simulink model "AFEC_model"  (R2024a)
settings: Solver=FixedStepAuto  StartTime=0.0  StopTime=7  FixedStep=1e-5  RelTol=1e-3
values from neighbouring files (symbols this model uses):
  C1 = 750e-6    (= 0.00075)    [scriptafec11.m]
  ka = Vdcref/2    (= 378.5)    [scriptafec11.m]
  kii_1 = 2*pi*fbi*r/ka    (= 0.014940202844)    [scriptafec11.m]
  kiw_1 = kpw_1 / (a_l^2 * tau_1l)    [scriptafec11.m]
  kpi_1 = 2*pi*fbi*l/ka    (= 0.015936216367)    [scriptafec11.m]
  kpw_1 = C1 / kl / a_l / tau_1l    [scriptafec11.m]
  l = 4.8e-3    (= 0.0048)    [scriptafec11.m]
  r = 0.0045    [scriptafec11.m]
  t_c = 1.5    [scriptafec11.m]
  t_pll = 1.3    [scriptafec11.m]
  t_precharge = 1    [scriptafec11.m]
  t_v = 1.75    [scriptafec11.m]
  tau_fl = 1 / 200    (= 0.005)    [scriptafec11.m]
  Vdcref = 757    [scriptafec11.m]
libraries: spsVoltageMeasurementLib x8, spsCurrentMeasurementLib x7, spsIGBTDiodeLib x6, spsSeriesRLCBranchLib x3, spsFirstOrderFilterLib x3, spsThreePhaseSeriesRLCBranchLib x2, spsControlledVoltageSourceLib x1, spsTriangleGeneratorLib x1, spsThreePhaseBreakerLib x1, spsThreePhaseSourceLib x1, sps_lib x1
settings Model: Creator=SSP Family  LastModifiedBy=khush
settings SolverCC: ZeroCrossAlgorithm=Adaptive
settings DebuggingCC: MaskedZcDiagnostic=none  IgnoredZcDiagnostic=none

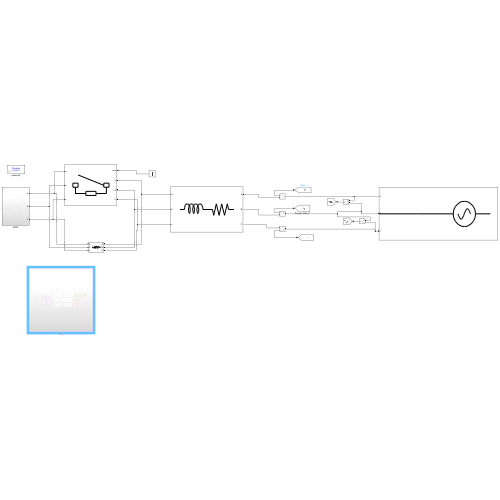
[thumbnail: Simulink's stored preview of the top-level diagram]
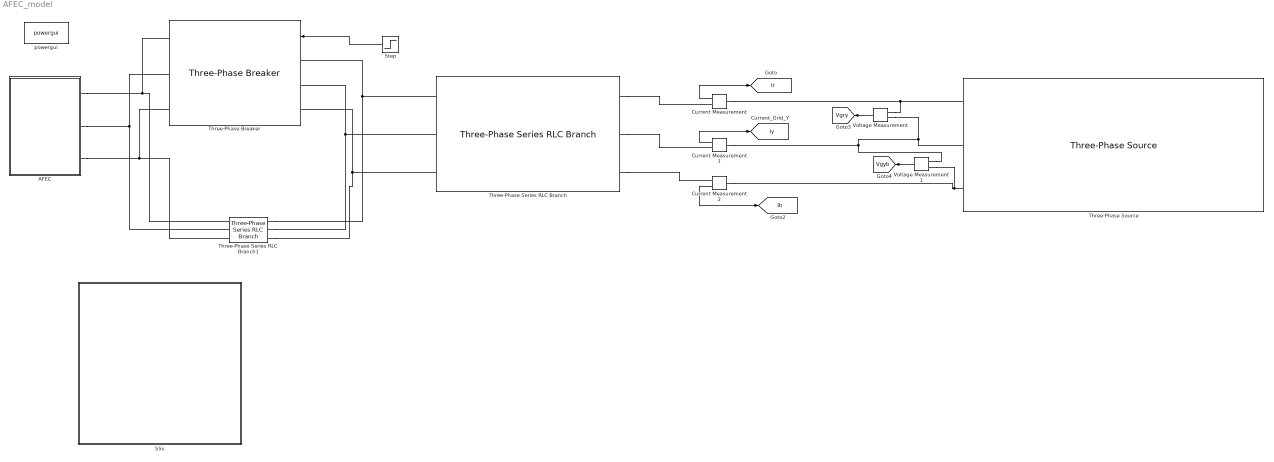
== system AFEC_model ==
  AFEC : Subsystem
  Current Measurement : spsCurrentMeasurementLib/Current Measurement  PhasorSimulation=off  OutputType=Complex  PSBequivalent=0
  Current Measurement1 : spsCurrentMeasurementLib/Current Measurement  PhasorSimulation=off  OutputType=Complex  PSBequivalent=0
  Current Measurement2 : spsCurrentMeasurementLib/Current Measurement  PhasorSimulation=off  OutputType=Complex  PSBequivalent=0
  SSs : Subsystem
  Step : Step  Time=t_precharge  SampleTime=0
  Three-Phase Series RLC Branch : spsThreePhaseSeriesRLCBranchLib/Three-Phase Series RLC Branch  LConnTagsString=A|B|C  RConnTagsString=A|B|C  BranchType=RL  Resistance=r  Inductance=l  Capacitance=1e-6  Measurements=None
  Three-Phase Series RLC Branch1 : spsThreePhaseSeriesRLCBranchLib/Three-Phase Series RLC Branch  LConnTagsString=A|B|C  RConnTagsString=A|B|C  BranchType=R  Resistance=2e3  Inductance=1e-3  Capacitance=1e-6  Measurements=None
  Three-Phase Breaker : spsThreePhaseBreakerLib/Three-Phase Breaker  InitialState=open  SwitchA=on  SwitchB=on  SwitchC=on  SwitchTimes="[1/60  5/60]"  External=on  BreakerResistance=0.01  SnubberResistance=1e6  SnubberCapacitance=inf  Measurements=None
  Three-Phase Source : spsThreePhaseSourceLib/Three-Phase Source  InternalConnection=Y  VoltagePhases=off  Voltage=400/sqrt(3)  PhaseAngle=0  Voltage_phases=[25e3 25e3 25e3]/sqrt(3)  PhaseAngles_phases=[0 -120 +120]  Frequency=50  NonIdealSource=off  SpecifyImpedance=off  Resistance=0  Inductance=0  ShortCircuitLevel=100e6  BaseVoltage=25e3  XRratio=7  BusType=swing  Pref=10e3  Qref=0  Prefabc=[10e3, 10e3, 10e3]  Qrefabc=[0, 0, 0]  Qmin=-inf  Qmax=inf
  Voltage Measurement : spsVoltageMeasurementLib/Voltage Measurement  PhasorSimulation=off  OutputType=Complex  PSBequivalent=0
  Voltage Measurement1 : spsVoltageMeasurementLib/Voltage Measurement  PhasorSimulation=off  OutputType=Complex  PSBequivalent=0
  powergui : sps_lib/powergui  Priority=1  SimulationMode=Discrete  SampleTime=1e-5  frequency=60  Iterations=50  frequencyindice=0  Pbase=100e6  ErrMax=1e-4  UnitsV=kV  UnitsW=MW  buscounter=0  FunctionMessages=off  echomessages=off  EnableUseOfTLC=off  CurrentSourceSwitches=off  DisableSnubberDevices=off  DisableRonSwitches=off  DisableVfSwitches=off  DisplayEquations=off  AutomaticDiscreteSolvers=off  SolverType=Tustin/Backward Euler (TBE)  Interpol=off  ExternalGateDelay=off  methode=off  Ts=100  x0status=blocks  SPID=on  SwTol=0  HookPort=off  NonlinearTolerance=1e-4  nMaxIteration=100  ContinueOnMaxIteration=off  RestoreLinks=warning  ResistiveCurrentMeasurement=off  Frange=[0:2:500]  Ylog=off  Xlog=on  ShowGrid=off  save=off  variable=ZData  structure=0  ZoomFFT=off  StartTime=0.0  cycles=1  DisplayStyle=1  fundamental=60  FreqAxis=off  MaxFrequency=1000  frequencyindicesteady=1  RmsSteady=1  display=off
  tag scope: Ib=global, Ir=global, Iy=global, Vgry=global, Vgyb=global
  wires:
  Current Measurement2/1 -> [Ib]
  Voltage Measurement/1 -> [Vgry]
  Voltage Measurement1/1 -> [Vgyb]
  Step/1 -> Three-Phase Breaker/1
  Current Measurement/1 -> [Ir]
  Current Measurement1/1 -> [Iy]
  connections:
  Current Measurement/LConn1 -- Three-Phase Source/RConn1 -- Voltage Measurement/LConn1
  Voltage Measurement1/LConn1 -- Voltage Measurement/LConn2 -- Three-Phase Source/RConn2 -- Current Measurement1/LConn1
  Voltage Measurement1/LConn2 -- Current Measurement2/LConn1 -- Three-Phase Source/RConn3
  Three-Phase Series RLC Branch1/LConn2 -- Three-Phase Series RLC Branch/RConn2 -- Three-Phase Breaker/LConn2
  Three-Phase Series RLC Branch1/LConn1 -- Three-Phase Series RLC Branch/RConn1 -- Three-Phase Breaker/LConn1
  Three-Phase Breaker/RConn1 -- Three-Phase Series RLC Branch1/RConn1 -- AFEC/LConn1
  Three-Phase Series RLC Branch1/LConn3 -- Three-Phase Series RLC Branch/RConn3 -- Three-Phase Breaker/LConn3
  Three-Phase Breaker/RConn3 -- Three-Phase Series RLC Branch1/RConn3 -- AFEC/LConn3
  Three-Phase Series RLC Branch1/RConn2 -- AFEC/LConn2 -- Three-Phase Breaker/RConn2
  Three-Phase Series RLC Branch/LConn1 -- Current Measurement/RConn1
  Three-Phase Series RLC Branch/LConn2 -- Current Measurement1/RConn1
  Three-Phase Series RLC Branch/LConn3 -- Current Measurement2/RConn1

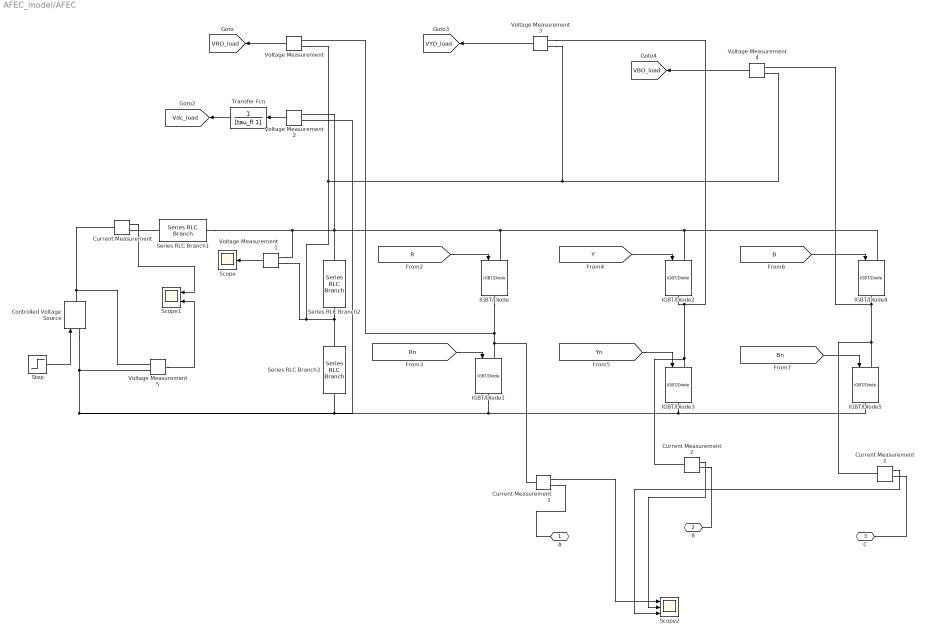
== system AFEC_model/AFEC ==
  Controlled Voltage Source : spsControlledVoltageSourceLib/Controlled Voltage Source  Initialize=on  Source_Type=DC  Amplitude=800  Phase=0  Frequency=0  Measurements=None
  Current Measurement{,1..3} (4 alike) : spsCurrentMeasurementLib/Current Measurement  PhasorSimulation=off  OutputType=Complex  PSBequivalent=0
  IGBT/Diode{,1..5} (6 alike) : spsIGBTDiodeLib/IGBT//Diode  Ron=1e-3  Rs=1e5  Cs=inf  Measurements=off
  Scope : Scope
  Scope1 : Scope  NumInputPorts=2
  Scope2 : Scope  NumInputPorts=3
  Series RLC Branch1 : spsSeriesRLCBranchLib/Series RLC Branch  LConnTagsString=__new0  RConnTagsString=__new0  BranchType=R  Resistance=10  Inductance=1e-3  SetiL0=off  InitialCurrent=0  Capacitance=1e-6  Setx0=off  InitialVoltage=0  Measurements=None
  Series RLC Branch2 : spsSeriesRLCBranchLib/Series RLC Branch  LConnTagsString=__new0  RConnTagsString=__new0  BranchType=C  Resistance=1  Inductance=1e-3  SetiL0=off  InitialCurrent=0  Capacitance=C1  Setx0=off  InitialVoltage=0  Measurements=None
  Series RLC Branch3 : spsSeriesRLCBranchLib/Series RLC Branch  LConnTagsString=__new0  RConnTagsString=__new0  BranchType=C  Resistance=1  Inductance=1e-3  SetiL0=off  InitialCurrent=0  Capacitance=C1  Setx0=off  InitialVoltage=0  Measurements=None
  Step : Step  After=800  SampleTime=0
  Transfer Fcn : TransferFcn  Denominator=[tau_fl 1]
  Voltage Measurement{,1..5} (6 alike) : spsVoltageMeasurementLib/Voltage Measurement  PhasorSimulation=off  OutputType=Complex  PSBequivalent=0
  A : PMIOPort  Side=Left
  B : PMIOPort  Port=2  Side=Left
  C : PMIOPort  Port=3  Side=Left
  tag scope: VBO_load=global, VRO_load=global, VYO_load=global, Vdc_load=global
  wires:
  Voltage Measurement4/1 -> [VBO_load]
  [Bn] -> IGBT/Diode5/1
  Voltage Measurement3/1 -> [VYO_load]
  Transfer Fcn/1 -> [Vdc_load]
  [B] -> IGBT/Diode4/1
  Voltage Measurement/1 -> [VRO_load]
  [Y] -> IGBT/Diode2/1
  Voltage Measurement2/1 -> Transfer Fcn/1
  [Rn] -> IGBT/Diode1/1
  [Yn] -> IGBT/Diode3/1
  [R] -> IGBT/Diode/1
  Step/1 -> Controlled Voltage Source/1
  Voltage Measurement1/1 -> Scope/1
  Voltage Measurement5/1 -> Scope1/2
  Current Measurement/1 -> Scope1/1
  Current Measurement1/1 -> Scope2/1
  Current Measurement2/1 -> Scope2/2
  Current Measurement3/1 -> Scope2/3
  connections:
  IGBT/Diode2/LConn1 -- Voltage Measurement1/LConn1 -- Series RLC Branch1/RConn1 -- Series RLC Branch2/LConn1 -- Voltage Measurement2/LConn1 -- IGBT/Diode/LConn1 -- IGBT/Diode4/LConn1
  IGBT/Diode/RConn1 -- Current Measurement1/LConn1 -- IGBT/Diode1/LConn1 -- Voltage Measurement/LConn1
  IGBT/Diode3/RConn1 -- IGBT/Diode5/RConn1 -- IGBT/Diode1/RConn1 -- Series RLC Branch3/RConn1 -- Controlled Voltage Source/LConn1 -- Voltage Measurement5/LConn2 -- Voltage Measurement2/LConn2
  IGBT/Diode2/RConn1 -- Voltage Measurement3/LConn1 -- Current Measurement2/LConn1 -- IGBT/Diode3/LConn1
  Voltage Measurement/LConn2 -- Voltage Measurement4/LConn2 -- Voltage Measurement3/LConn2 -- Voltage Measurement1/LConn2 -- Series RLC Branch2/RConn1 -- Series RLC Branch3/LConn1
  Controlled Voltage Source/RConn1 -- Current Measurement/LConn1 -- Voltage Measurement5/LConn1
  Current Measurement/RConn1 -- Series RLC Branch1/LConn1
  Voltage Measurement4/LConn1 -- Current Measurement3/LConn1 -- IGBT/Diode5/LConn1 -- IGBT/Diode4/RConn1
  Current Measurement1/RConn1 -- A/RConn1
  Current Measurement2/RConn1 -- B/RConn1
  Current Measurement3/RConn1 -- C/RConn1

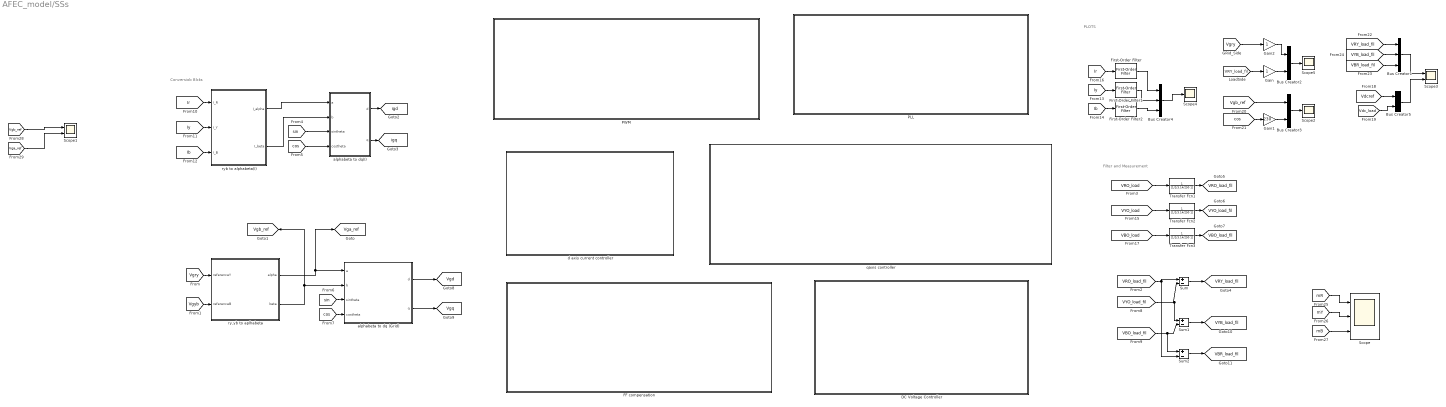
== system AFEC_model/SSs ==
  note: Conversiob Blcks
  note: PLOTS
  note: Filter and Measurement
  Bus Creator1 : BusCreator  Inputs=3
  Bus Creator2 : BusCreator  Inputs=2
  Bus Creator3 : BusCreator  Inputs=2
  Bus Creator4 : BusCreator  Inputs=3
  Bus Creator5 : BusCreator  Inputs=2
  DC Voltage Controller : Subsystem
  FF compensation : Subsystem
  First-Order Filter : spsFirstOrderFilterLib/First-Order Filter  FilterType=Lowpass  Tc=1e-3  Ts=0  Initialize=off  Vac_Init=[0, 0, 60]  Vdc_Init=0  PlotResponse=off  FreqRange="[0,  200,  1]"
  First-Order Filter1 : spsFirstOrderFilterLib/First-Order Filter  FilterType=Lowpass  Tc=10e-3  Ts=0  Initialize=off  Vac_Init=[0, 0, 60]  Vdc_Init=0  PlotResponse=off  FreqRange="[0,  200,  1]"
  First-Order Filter2 : spsFirstOrderFilterLib/First-Order Filter  FilterType=Lowpass  Tc=10e-3  Ts=0  Initialize=off  Vac_Init=[0, 0, 60]  Vdc_Init=0  PlotResponse=off  FreqRange="[0,  200,  1]"
  Gain : Gain
  Gain1 : Gain  Gain=230
  Gain2 : Gain
  PLL : Subsystem
  PWM : Subsystem
  Scope : Scope  NumInputPorts=3
  Scope1 : Scope  NumInputPorts=2
  Scope2 : Scope
  Scope3 : Scope  NumInputPorts=2
  Scope4 : Scope
  Scope5 : Scope
  Sum : Sum  Inputs=+-
  Sum1 : Sum  Inputs=+-
  Sum2 : Sum  Inputs=+-
  Transfer Fcn1 : TransferFcn  Denominator=[1/2/3.14/250 1]
  Transfer Fcn2 : TransferFcn  Denominator=[1/2/3.14/250 1]
  Transfer Fcn3 : TransferFcn  Denominator=[1/2/3.14/250 1]
  alphabeta to dq (Grid) : MATLAB Function  TreatAsAtomicUnit=on
  alphabeta to dq(I) : MATLAB Function  TreatAsAtomicUnit=on
  d axis current controller : Subsystem
  qaxis controller : Subsystem
  ry,yb to aplhabeta : MATLAB Function  TreatAsAtomicUnit=on
  ryb to alphabeta(I) : MATLAB Function  TreatAsAtomicUnit=on
  tag scope: VBO_load_fil=global, VBR_load_fil=global, VRO_load_fil=global, VRY_load_fil=global, VYB_load_fil=global, VYO_load_fil=global, Vga_ref=global, Vgb_ref=global, Vgd=global, Vgq=global, igd=global, igq=global
  wires:
  ry,yb to aplhabeta/2(beta) -> [Vgb_ref], alphabeta to dq (Grid)/2(b)
  [Ib] -> ryb to alphabeta(I)/3(I_B)
  ry,yb to aplhabeta/1(alpha) -> [Vga_ref], alphabeta to dq (Grid)/1(a)
  ryb to alphabeta(I)/1(I_alpha) -> alphabeta to dq(I)/1(a)
  [cos] -> alphabeta to dq (Grid)/4(costheta)
  [Vgry] -> ry,yb to aplhabeta/1(referenceY)
  alphabeta to dq(I)/1(d) -> [igd]
  [Iy] -> ryb to alphabeta(I)/2(I_Y)
  [cos] -> alphabeta to dq(I)/4(costheta)
  [sin] -> alphabeta to dq (Grid)/3(sintheta)
  [Ir] -> ryb to alphabeta(I)/1(I_R)
  [sin] -> alphabeta to dq(I)/3(sintheta)
  alphabeta to dq (Grid)/1(d) -> [Vgd]
  [Vgyb] -> ry,yb to aplhabeta/2(referenceB)
  alphabeta to dq(I)/2(q) -> [igq]
  alphabeta to dq (Grid)/2(q) -> [Vgq]
  ryb to alphabeta(I)/2(I_beta) -> alphabeta to dq(I)/2(b)
  [VBO_load] -> Transfer Fcn3/1
  Sum/1 -> [VRY_load_fil]
  [Iy] -> First-Order Filter1/1
  [VRY_load_fil] -> Gain/1
  Bus Creator3/1 -> Scope2/1
  Sum2/1 -> [VBR_load_fil]
  [Vgb_ref] -> Bus Creator3/1
  [cos] -> Gain1/1
  Sum1/1 -> [VYB_load_fil]
  Gain1/1 -> Bus Creator3/2
  Gain2/1 -> Bus Creator2/1
  Bus Creator2/1 -> Scope5/1
  First-Order Filter1/1 -> Bus Creator4/2
  [VRO_load] -> Transfer Fcn1/1
  Transfer Fcn1/1 -> [VRO_load_fil]
  [VRO_load_fil] -> Sum2/2, Sum/1
  [VYO_load] -> Transfer Fcn2/1
  Transfer Fcn3/1 -> [VBO_load_fil]
  Transfer Fcn2/1 -> [VYO_load_fil]
  Bus Creator4/1 -> Scope4/1
  [Ib] -> First-Order Filter2/1
  First-Order Filter/1 -> Bus Creator4/1
  [Ir] -> First-Order Filter/1
  [VYO_load_fil] -> Sum1/1, Sum/2
  Gain/1 -> Bus Creator2/2
  [VBO_load_fil] -> Sum2/1, Sum1/2
  First-Order Filter2/1 -> Bus Creator4/3
  [Vgry] -> Gain2/1
  Bus Creator1/1 -> Scope3/1
  [VBR_load_fil] -> Bus Creator1/3
  [Vdcref] -> Bus Creator5/1
  [VRY_load_fil] -> Bus Creator1/1
  [Vdc_load] -> Bus Creator5/2
  [VYB_load_fil] -> Bus Creator1/2
  Bus Creator5/1 -> Scope3/2
  [mR] -> Scope/1
  [mY] -> Scope/2
  [mB] -> Scope/3
  [Vgb_ref] -> Scope1/1
  [Vga_ref] -> Scope1/2

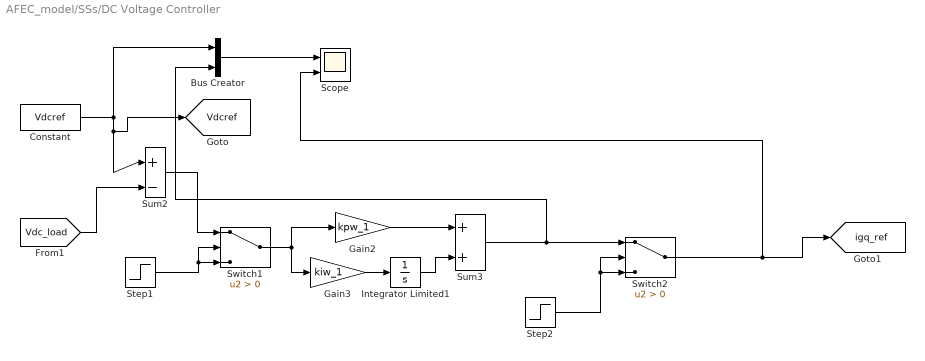
== system AFEC_model/SSs/DC Voltage Controller ==
  Bus Creator : BusCreator  Inputs=2
  Constant : Constant  Value=Vdcref
  Gain2 : Gain  Gain=kpw_1
  Gain3 : Gain  Gain=kiw_1
  Integrator Limited1 : Integrator  LimitOutput=on  UpperSaturationLimit=1  LowerSaturationLimit=0
  Scope : Scope  NumInputPorts=2
  Step1 : Step  Time=t_c  SampleTime=0
  Step2 : Step  Time=t_c  SampleTime=0
  Sum2 : Sum  Inputs=|+-
  Sum3 : Sum
  Switch1 : Switch  Criteria=u2 > Threshold  SaturateOnIntegerOverflow=off  InputSameDT=off
  Switch2 : Switch  Criteria=u2 > Threshold  SaturateOnIntegerOverflow=off  InputSameDT=off
  tag scope: Vdcref=global, igq_ref=global
  wires:
  Switch2/1 -> Scope/2, [igq_ref]
  Bus Creator/1 -> Scope/1
  Sum2/1 -> Switch1/1
  Gain3/1 -> Integrator Limited1/1
  Gain2/1 -> Sum3/1
  Step1/1 -> Switch1/3, Switch1/2
  Sum3/1 -> Bus Creator/2, Switch2/1
  Step2/1 -> Switch2/3, Switch2/2
  Switch1/1 -> Gain3/1, Gain2/1
  [Vdc_load] -> Sum2/2
  Integrator Limited1/1 -> Sum3/2
  Constant/1 -> Sum2/1, [Vdcref], Bus Creator/1

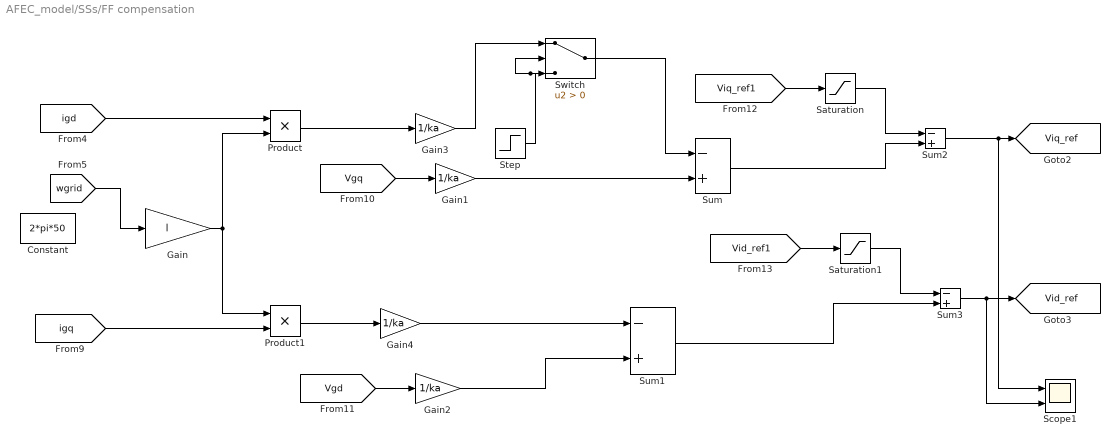
== system AFEC_model/SSs/FF compensation ==
  Constant : Constant  Value=2*pi*50
  Gain : Gain  Gain=l
  Gain{1..4} (4 alike) : Gain  Gain=1/ka
  Product : Product
  Product1 : Product
  Saturation : Saturate  UpperLimit=1  LowerLimit=-1
  Saturation1 : Saturate  UpperLimit=1  LowerLimit=-1
  Scope1 : Scope  NumInputPorts=2
  Step : Step  Time=t_c  SampleTime=0
  Sum{,1..3} (4 alike) : Sum  Inputs=-+
  Switch : Switch  Criteria=u2 > Threshold  SaturateOnIntegerOverflow=off  InputSameDT=off
  tag scope: Vid_ref=global, Viq_ref=global
  wires:
  Sum3/1 -> Scope1/2, [Vid_ref]
  Gain2/1 -> Sum1/2
  [Vgd] -> Gain2/1
  Step/1 -> Switch/2, Switch/3
  Sum/1 -> Sum2/2
  Gain/1 -> Product1/1, Product/2
  Gain1/1 -> Sum/2
  Saturation/1 -> Sum2/1
  Sum2/1 -> Scope1/1, [Viq_ref]
  [Viq_ref1] -> Saturation/1
  [igd] -> Product/1
  Saturation1/1 -> Sum3/1
  [Vgq] -> Gain1/1
  Sum1/1 -> Sum3/2
  Gain3/1 -> Switch/1
  [Vid_ref1] -> Saturation1/1
  Product/1 -> Gain3/1
  Product1/1 -> Gain4/1
  Switch/1 -> Sum/1
  Gain4/1 -> Sum1/1
  [igq] -> Product1/2
  [wgrid] -> Gain/1

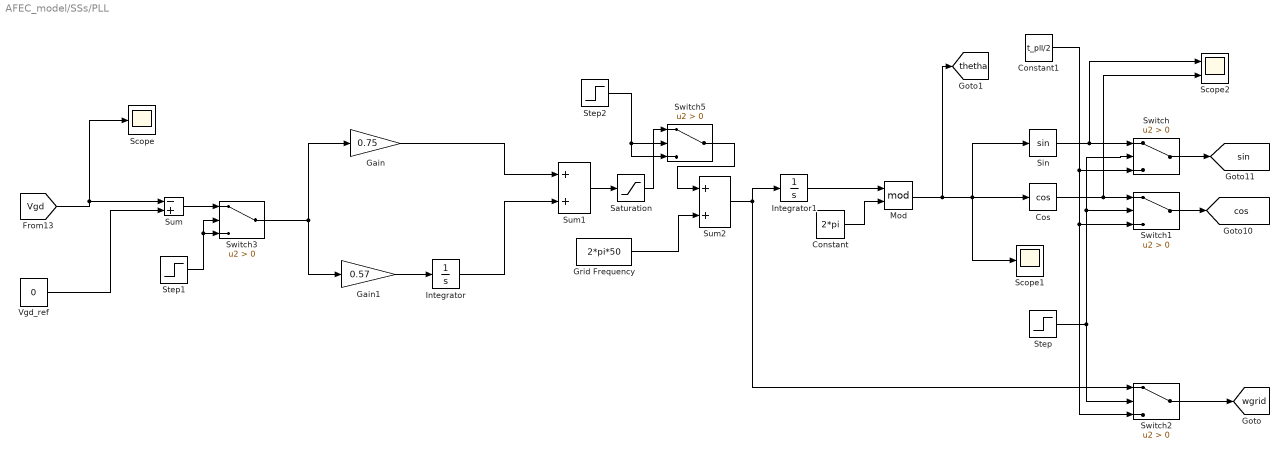
== system AFEC_model/SSs/PLL ==
  Constant : Constant  Value=2*pi
  Constant1 : Constant  Value=t_pll/2
  Cos : Trigonometry  Operator=cos
  Gain : Gain  Gain=0.75
  Gain1 : Gain  Gain=0.57
  Grid Frequency : Constant  Value=2*pi*50
  Integrator : Integrator  LimitOutput=on  UpperSaturationLimit=2*pi*50  LowerSaturationLimit=-2*pi*50
  Integrator1 : Integrator
  Mod : Math  Operator=mod
  Saturation : Saturate  UpperLimit=2*pi*50  LowerLimit=-2*pi*50
  Scope : Scope
  Scope1 : Scope
  Scope2 : Scope  NumInputPorts=2
  Sin : Trigonometry
  Step : Step  Time=t_pll  SampleTime=0
  Step1 : Step  Time=t_pll  SampleTime=0
  Step2 : Step  Time=t_pll  SampleTime=0
  Sum : Sum  Inputs=-+
  Sum1 : Sum
  Sum2 : Sum
  Switch{,1..3,5} (5 alike) : Switch  Criteria=u2 > Threshold  SaturateOnIntegerOverflow=off  InputSameDT=off
  Vgd_ref : Constant  Value=0
  tag scope: cos=global, sin=global, thetha=global, wgrid=global
  wires:
  Gain1/1 -> Integrator/1
  Constant/1 -> Mod/2
  Gain/1 -> Sum1/1
  Grid Frequency/1 -> Sum2/2
  Sum2/1 -> Integrator1/1, Switch2/1
  Sum1/1 -> Saturation/1
  Integrator/1 -> Sum1/2
  Integrator1/1 -> Mod/1
  Vgd_ref/1 -> Sum/2
  Mod/1 -> [thetha], Cos/1, Sin/1, Scope1/1
  [Vgd] -> Scope/1, Sum/1
  Switch/1 -> [sin]
  Switch1/1 -> [cos]
  Switch2/1 -> [wgrid]
  Sin/1 -> Scope2/1, Switch/1
  Cos/1 -> Scope2/2, Switch1/1
  Constant1/1 -> Switch2/3, Switch1/3, Switch/3
  Step/1 -> Switch2/2, Switch1/2, Switch/2
  Sum/1 -> Switch3/1
  Switch3/1 -> Gain1/1, Gain/1
  Step1/1 -> Switch3/2, Switch3/3
  Saturation/1 -> Switch5/1
  Switch5/1 -> Sum2/1
  Step2/1 -> Switch5/3, Switch5/2

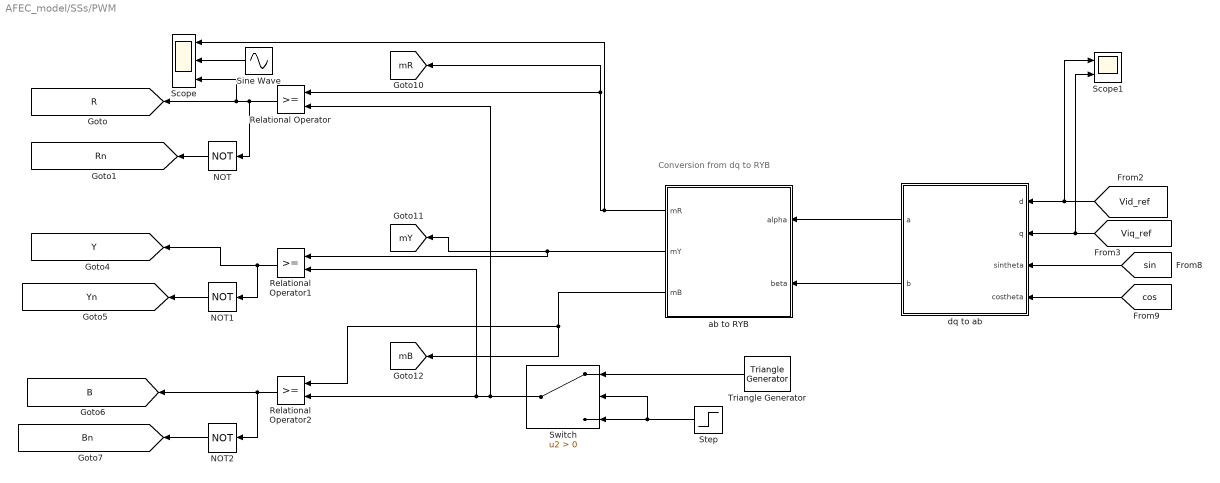
== system AFEC_model/SSs/PWM ==
  note: Conversion from dq to RYB
  NOT : Logic  Operator=NOT  IconShape=distinctive  AllPortsSameDT=off  OutDataTypeStr=boolean
  NOT1 : Logic  Operator=NOT  IconShape=distinctive  AllPortsSameDT=off  OutDataTypeStr=boolean
  NOT2 : Logic  Operator=NOT  IconShape=distinctive  AllPortsSameDT=off  OutDataTypeStr=boolean
  Relational Operator : RelationalOperator  OutDataTypeStr=boolean  RndMeth=Simplest  InputSameDT=off
  Relational Operator1 : RelationalOperator  OutDataTypeStr=boolean  RndMeth=Simplest  InputSameDT=off
  Relational Operator2 : RelationalOperator  OutDataTypeStr=boolean  RndMeth=Simplest  InputSameDT=off
  Scope : Scope  NumInputPorts=3
  Scope1 : Scope  NumInputPorts=2
  Sine Wave : Sin  Frequency=50*2*pi  SampleTime=0
  Step : Step  Time=t_v  SampleTime=0
  Switch : Switch  Criteria=u2 > Threshold  SaturateOnIntegerOverflow=off  InputSameDT=off
  Triangle Generator : spsTriangleGeneratorLib/Triangle Generator  Freq=fsw_1  Phase=90  Ts=0
  ab to RYB : MATLAB Function  TreatAsAtomicUnit=on
  dq to ab : MATLAB Function  TreatAsAtomicUnit=on
  tag scope: B=global, Bn=global, R=global, Rn=global, Y=global, Yn=global, mB=global, mR=global, mY=global
  wires:
  Relational Operator1/1 -> [Y], NOT1/1
  NOT1/1 -> [Yn]
  Relational Operator/1 -> Scope/3, [R], NOT/1
  NOT/1 -> [Rn]
  Relational Operator2/1 -> NOT2/1, [B]
  NOT2/1 -> [Bn]
  Triangle Generator/1 -> Switch/1
  Switch/1 -> Relational Operator1/2, Relational Operator2/2, Relational Operator/2
  Step/1 -> Switch/2, Switch/3
  Sine Wave/1 -> Scope/2
  ab to RYB/1(mR) -> [mR], Relational Operator/1, Scope/1
  ab to RYB/3(mB) -> Relational Operator2/1, [mB]
  ab to RYB/2(mY) -> Relational Operator1/1, [mY]
  [sin] -> dq to ab/3(sintheta)
  [Vid_ref] -> Scope1/1, dq to ab/1(d)
  [Viq_ref] -> Scope1/2, dq to ab/2(q)
  dq to ab/1(a) -> ab to RYB/1(alpha)
  dq to ab/2(b) -> ab to RYB/2(beta)
  [cos] -> dq to ab/4(costheta)

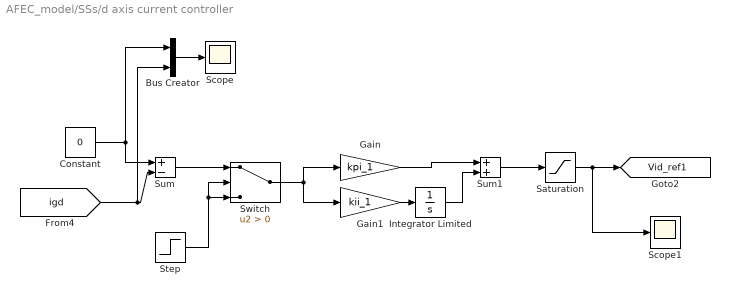
== system AFEC_model/SSs/d axis current controller ==
  Bus Creator : BusCreator  Inputs=2
  Constant : Constant  Value=0
  Gain : Gain  Gain=kpi_1
  Gain1 : Gain  Gain=kii_1
  Integrator Limited : Integrator  LimitOutput=on  UpperSaturationLimit=1  LowerSaturationLimit=0
  Saturation : Saturate  UpperLimit=1  LowerLimit=-1
  Scope : Scope
  Scope1 : Scope
  Step : Step  Time=t_pll  SampleTime=0
  Sum : Sum  Inputs=+-
  Sum1 : Sum
  Switch : Switch  Criteria=u2 > Threshold  SaturateOnIntegerOverflow=off  InputSameDT=off
  tag scope: Vid_ref1=global
  wires:
  Constant/1 -> Sum/1, Bus Creator/1
  Gain1/1 -> Integrator Limited/1
  Bus Creator/1 -> Scope/1
  Switch/1 -> Gain/1, Gain1/1
  Integrator Limited/1 -> Sum1/2
  Saturation/1 -> Scope1/1, [Vid_ref1]
  Sum/1 -> Switch/1
  Gain/1 -> Sum1/1
  Step/1 -> Switch/3, Switch/2
  Sum1/1 -> Saturation/1
  [igd] -> Bus Creator/2, Sum/2

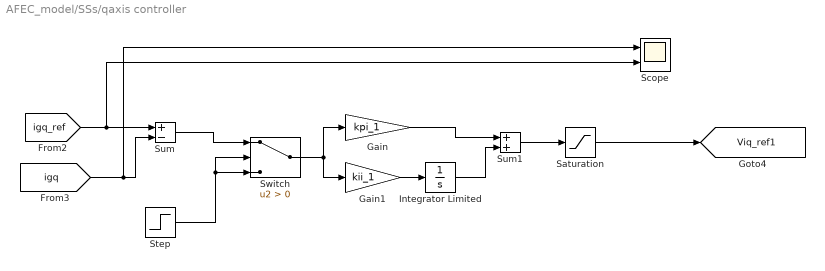
== system AFEC_model/SSs/qaxis controller ==
  Gain : Gain  Gain=kpi_1
  Gain1 : Gain  Gain=kii_1
  Integrator Limited : Integrator  LimitOutput=on  UpperSaturationLimit=1.5  LowerSaturationLimit=-1.5
  Saturation : Saturate  UpperLimit=1  LowerLimit=-1
  Scope : Scope  NumInputPorts=2
  Step : Step  Time=t_pll  SampleTime=0
  Sum : Sum  Inputs=+-
  Sum1 : Sum
  Switch : Switch  Criteria=u2 > Threshold  SaturateOnIntegerOverflow=off  InputSameDT=off
  tag scope: Viq_ref1=global
  wires:
  Switch/1 -> Gain/1, Gain1/1
  [igq_ref] -> Scope/2, Sum/1
  Saturation/1 -> [Viq_ref1]
  Step/1 -> Switch/3, Switch/2
  Sum/1 -> Switch/1
  Gain1/1 -> Integrator Limited/1
  Sum1/1 -> Saturation/1
  Gain/1 -> Sum1/1
  [igq] -> Scope/1, Sum/2
  Integrator Limited/1 -> Sum1/2

== matlab function AFEC_model/SSs/alphabeta to dq(I) ==
  data: a input; d output; b input; sintheta input; costheta input; q output
function [d, q] = fcn(a, b, sintheta, costheta)
    d = a * costheta + b * sintheta;
    q = -a * sintheta + b * costheta;
end

== matlab function AFEC_model/SSs/alphabeta to dq (Grid) ==
  data: a input; d output; b input; sintheta input; costheta input; q output
function [d, q] = fcn(a, b, sintheta, costheta)
    d = a * costheta + b * sintheta;
    q = -a * sintheta + b * costheta;
end

== matlab function AFEC_model/SSs/ryb to alphabeta(I) ==
  data: I_R input; I_Y input; I_B input; I_alpha output; I_beta output
function [I_alpha, I_beta] = fcn(I_R, I_Y, I_B)
    I_alpha = (2/3) * I_R - (1/3) * (I_Y + I_B);
    I_beta = (1/sqrt(3)) * (I_Y - I_B);
end

== matlab function AFEC_model/SSs/ry,yb to aplhabeta ==
  data: alpha output; beta output; referenceY input; referenceB input
function [alpha, beta] = fcn(referenceY, referenceB)
    alpha = (2/3) * (0 - 0.5 * (referenceY + referenceB));
    beta = (1/sqrt(3)) * (referenceY - referenceB);
end

== matlab function AFEC_model/SSs/PWM/ab to RYB ==
  data: alpha input; mR output; beta input; mY output; mB output
function [mR, mY, mB] = fcn(alpha, beta)
    mR = (2/3) * alpha;
    mY = (-1/3) * alpha + (1/sqrt(3)) * beta;
    mB = (-1/3) * alpha - (1/sqrt(3)) * beta;
end

== matlab function AFEC_model/SSs/PWM/dq to ab ==
  data: d input; a output; b output; q input; sintheta input; costheta input
function [a, b] = fcn(d, q, sintheta, costheta)
    a = d * costheta - q * sintheta;
    b = d * sintheta + q * costheta;
end
